simulink model "WindFarmGFMControl"  (R2025b)
settings: Solver=VariableStepAuto  StartTime=0.0  StopTime=Tsim  FixedStep=Ts  MaxStep=1  MinStep=Ts  RelTol=1e-3
PreLoadFcn:
  | run('WindFarmGFMControlParameters.m')
undefined symbols (not defined in the file): DiscIntNeverNeededParam, feeder, frt, gGFM, grid, line, loads, lvrt, mGFM, pmsm, time, Ts, windController, windTransformer, windTurbine
libraries: ee_lib x21, nesl_utility x14, eeGeneralControl x4, fl_lib x3, eeTransforms x2, eePowerMeasurement x1, eeSinusoidalMeasurementV2 x1
(part 2 of 2)

== system WindFarmGFMControl/Loads/CB1 ==
  Input : Inport
  Circuit Breaker Step off3 : ee_lib/Switches & Breakers/Circuit Breaker (Three-Phase)  R_closed=0.001 Ohm  G_open=1e-4 1/Ohm  threshold=0.5 V  breaker_behavior=ee.enum.switches.breakerBehavior.zeroCrossingDisable
      settings: InternalSimscapePortConfiguration="{\"Bottom\":[],\"Left\":[{\"id\":\"vT\",\"label\":\"vT\",\"type\":\"input\"},{\"id\":\"N1\",\"label\":\"~1\",\"type\":\"foundation.electrical.three_phase\"}],\"Right\":[{\"id\":\"N2\",\"label\":\"~2\",\"type\":\"foundation.electrical.three_phase\"}],\"Top\":[]}"
  Simulink-PS Converter3 : nesl_utility/Simulink-PS Converter  PhysicalDomain=network_engine_domain  SubClassName=ps_input  LeftPortType=input  RightPortType=output  PseudoPeriodic=off  Frequencies=[]  NoiseDistribution=none  NoiseParameters=[]  Unit=1  AffineConversion=off  FilteringAndDerivatives=zero  SimscapeFilterOrder=1  InputFilterTimeConstant=0.001  UdotUserProvided=1
  Conn2 : PMIOPort  Side=Left
  Conn1 : PMIOPort  Port=2  Side=Right
  wires:
  Input/1 -> Simulink-PS Converter3/1
  connections:
  Circuit Breaker Step off3/RConn1 -- Conn1/RConn1
  Circuit Breaker Step off3/LConn1 -- Simulink-PS Converter3/RConn1
  Circuit Breaker Step off3/LConn2 -- Conn2/RConn1

== system WindFarmGFMControl/PLL & Measurements/Measurement1 ==
  u : Inport
  Ig : Outport
  wires:
  u/1 -> Ig/1

== system WindFarmGFMControl/PLL & Measurements/Measurement2 ==
  u : Inport
  Vg : Outport
  wires:
  u/1 -> Vg/1

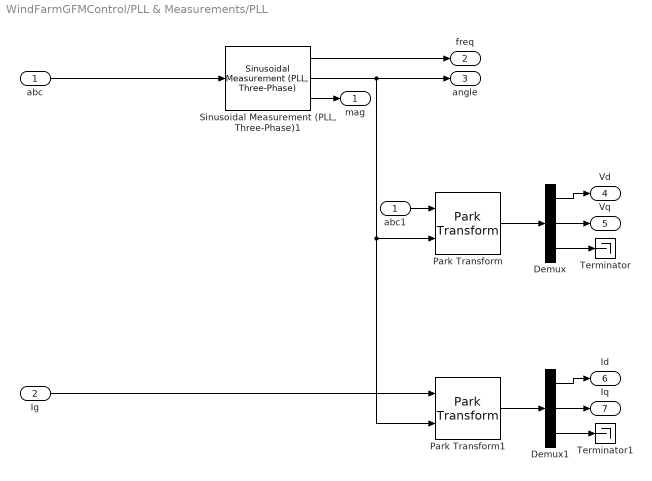
== system WindFarmGFMControl/PLL & Measurements/PLL ==
  abc : Inport
  Ig : Inport  Port=2
  Demux : Demux  Outputs=3
  Demux1 : Demux  Outputs=3
  Park Transform : eeTransforms/Park Transform  AxisAlignment=Q-axis  PowerInvariant=off
  Park Transform1 : eeTransforms/Park Transform  AxisAlignment=Q-axis  PowerInvariant=off
  "Sinusoidal Measurement (PLL, Three-Phase)1" : eeSinusoidalMeasurementV2/Sinusoidal Measurement (PLL, Three-Phase)  InputFilter=on  InputNormalization=off  Kp_LF=pll.kp  Ki_LF=pll.ki  F0=grid.frequency  Theta0=0  Ts=Ts
      settings: LibrarySourceBlock=|
      | ee_sl_lib/Measurements/Sinusoidal Measurement
      | (PLL, Three-Phase)
  Terminator : Terminator
  Terminator1 : Terminator
  abc1 : InportShadow
  mag : Outport
  freq : Outport  Port=2
  angle : Outport  Port=3
  Vd : Outport  Port=4
  Vq : Outport  Port=5
  Id : Outport  Port=6
  Iq : Outport  Port=7
  wires:
  Demux/3 -> Terminator/1
  Park Transform/1 -> Demux/1
  Demux/1 -> Vd/1
  Demux/2 -> Vq/1
  "Sinusoidal Measurement (PLL, Three-Phase)1"/3 -> mag/1
  "Sinusoidal Measurement (PLL, Three-Phase)1"/2 -> angle/1, Park Transform/2, Park Transform1/2
  Ig/1 -> Park Transform1/1
  Demux1/2 -> Iq/1
  Park Transform1/1 -> Demux1/1
  Demux1/1 -> Id/1
  Demux1/3 -> Terminator1/1
  abc1/1 -> Park Transform/1
  abc/1 -> "Sinusoidal Measurement (PLL, Three-Phase)1"/1
  "Sinusoidal Measurement (PLL, Three-Phase)1"/1 -> freq/1

== system WindFarmGFMControl/Wind Farm/CB2 ==
  Input : Inport
  Circuit Breaker Step off3 : ee_lib/Switches & Breakers/Circuit Breaker (Three-Phase)  R_closed=0.001 Ohm  G_open=1e-4 1/Ohm  threshold=0.5 V  breaker_behavior=ee.enum.switches.breakerBehavior.zeroCrossingDisable
      settings: InternalSimscapePortConfiguration="{\"Bottom\":[],\"Left\":[{\"id\":\"vT\",\"label\":\"vT\",\"type\":\"input\"},{\"id\":\"N1\",\"label\":\"~1\",\"type\":\"foundation.electrical.three_phase\"}],\"Right\":[{\"id\":\"N2\",\"label\":\"~2\",\"type\":\"foundation.electrical.three_phase\"}],\"Top\":[]}"
  Simulink-PS Converter3 : nesl_utility/Simulink-PS Converter  PhysicalDomain=network_engine_domain  SubClassName=ps_input  LeftPortType=input  RightPortType=output  PseudoPeriodic=off  Frequencies=[]  NoiseDistribution=none  NoiseParameters=[]  Unit=1  AffineConversion=off  FilteringAndDerivatives=zero  SimscapeFilterOrder=1  InputFilterTimeConstant=0.001  UdotUserProvided=1
  Conn2 : PMIOPort  Side=Left
  Conn1 : PMIOPort  Port=2  Side=Right
  wires:
  Input/1 -> Simulink-PS Converter3/1
  connections:
  Circuit Breaker Step off3/RConn1 -- Conn1/RConn1
  Circuit Breaker Step off3/LConn1 -- Simulink-PS Converter3/RConn1
  Circuit Breaker Step off3/LConn2 -- Conn2/RConn1

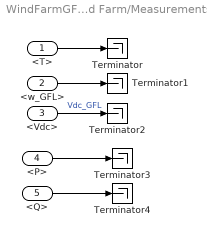
== system WindFarmGFMControl/Wind Farm/Measurements ==
  <T> : Inport
  <w_GFL> : Inport  Port=2
  <Vdc> : Inport  Port=3
  <P> : Inport  Port=4
  <Q> : Inport  Port=5
  Terminator{,1..4} (5 alike) : Terminator
  wires:
  <Vdc>/1 -> Terminator2/1  "Vdc_GFL"
  <Q>/1 -> Terminator4/1
  <w_GFL>/1 -> Terminator1/1
  <T>/1 -> Terminator/1
  <P>/1 -> Terminator3/1

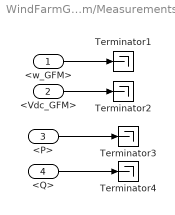
== system WindFarmGFMControl/Wind Farm/Measurements1 ==
  <w_GFM> : Inport
  <Vdc_GFM> : Inport  Port=2
  <P> : Inport  Port=3
  <Q> : Inport  Port=4
  Terminator{1..4} (4 alike) : Terminator
  wires:
  <P>/1 -> Terminator3/1
  <w_GFM>/1 -> Terminator1/1
  <Q>/1 -> Terminator4/1
  <Vdc_GFM>/1 -> Terminator2/1

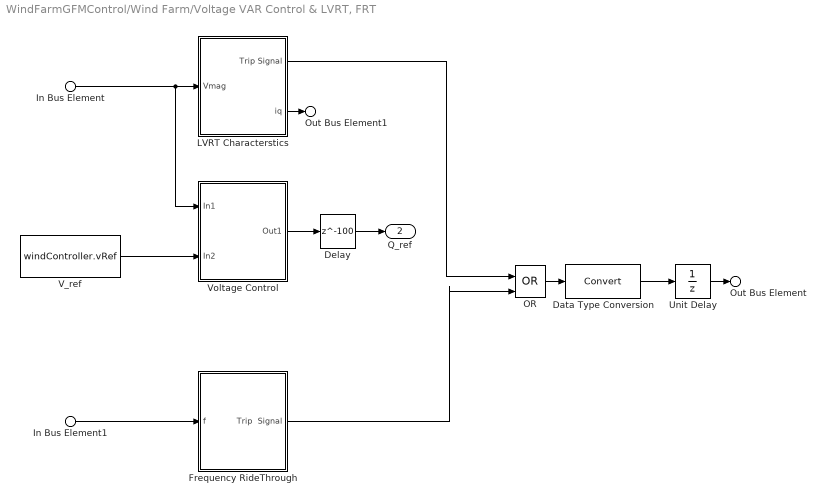
== system WindFarmGFMControl/Wind Farm/Voltage VAR Control & LVRT, FRT ==
  In Bus Element : Inport  PortName=Vbus  Element=Vmag
  In Bus Element1 : Inport  PortName=Vbus  Element=w
  Data Type Conversion : DataTypeConversion  RndMeth=Nearest  SaturateOnIntegerOverflow=off
  Delay : Delay  DelayLength=100
  Frequency RideThrough : Subsystem
  LVRT Characterstics : Subsystem
  OR : Logic  Operator=OR  IconShape=distinctive  AllPortsSameDT=off  OutDataTypeStr=boolean
  Unit Delay : UnitDelay  SampleTime=-1  HasFrameUpgradeWarning=on
  V_ref : Constant  Value=windController.vRef  SampleTime=Ts
  Voltage Control : Subsystem
  Out Bus Element : Outport  PortName=LVRT  Element=breaker
  Out Bus Element1 : Outport  PortName=LVRT  Element=iq
  Q_ref : Outport  Port=2
  wires:
  In Bus Element/1 -> LVRT Characterstics/1(Vmag), Voltage Control/1(In1)
  LVRT Characterstics/2(iq) -> Out Bus Element1/1
  V_ref/1 -> Voltage Control/2(In2)
  Voltage Control/1(Out1) -> Delay/1
  OR/1 -> Data Type Conversion/1
  LVRT Characterstics/1(Trip Signal) -> OR/1
  In Bus Element1/1 -> Frequency RideThrough/1(f)
  Data Type Conversion/1 -> Unit Delay/1
  Frequency RideThrough/1(Trip  Signal) -> OR/2
  Unit Delay/1 -> Out Bus Element/1
  Delay/1 -> Q_ref/1

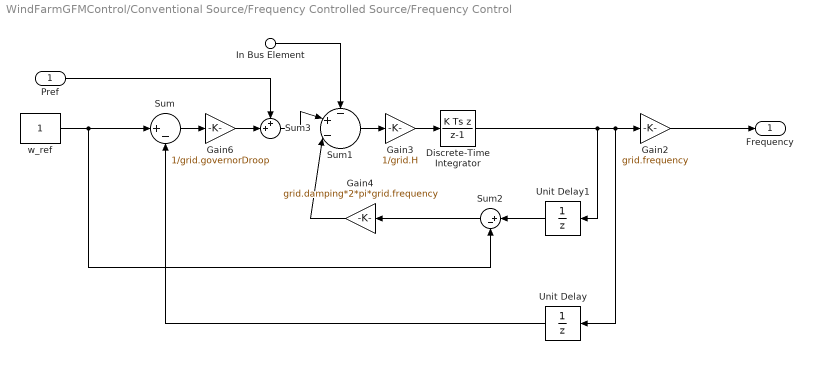
== system WindFarmGFMControl/Conventional Source/Frequency Controlled Source/Frequency Control ==
  Pref : Inport
  In Bus Element : Inport  Port=2  PortName=Grid  Element=Pe
  Discrete-Time Integrator : DiscreteIntegrator  IntegratorMethod=Integration: Backward Euler  InitialCondition=1  SampleTime=Ts  LimitOutput=on  UpperSaturationLimit=1.1  LowerSaturationLimit=0.9  ICPrevOutput=DiscIntNeverNeededParam  ICPrevScaledInput=DiscIntNeverNeededParam
  Gain2 : Gain  Gain=grid.frequency
  Gain3 : Gain  Gain=1/grid.H
  Gain4 : Gain  Gain=grid.damping*2*pi*grid.frequency
  Gain6 : Gain  Gain=1/grid.governorDroop
  Sum : Sum  Inputs=|+-
  Sum1 : Sum  Inputs=-+-|
  Sum2 : Sum  Inputs=|+-
  Sum3 : Sum  Inputs=++|
  Unit Delay : UnitDelay  InitialCondition=1  SampleTime=grid.sensorTime  HasFrameUpgradeWarning=on
  Unit Delay1 : UnitDelay  InitialCondition=1  SampleTime=grid.sensorTime  HasFrameUpgradeWarning=on
  w_ref : Constant
  Frequency : Outport
  wires:
  Sum3/1 -> Sum1/2
  w_ref/1 -> Sum2/2, Sum/1
  Sum1/1 -> Gain3/1
  Gain3/1 -> Discrete-Time Integrator/1
  Gain6/1 -> Sum3/2
  Gain2/1 -> Frequency/1
  Sum2/1 -> Gain4/1
  Sum/1 -> Gain6/1
  Pref/1 -> Sum3/1
  Gain4/1 -> Sum1/3
  In Bus Element/1 -> Sum1/1
  Discrete-Time Integrator/1 -> Unit Delay1/1, Unit Delay/1, Gain2/1
  Unit Delay/1 -> Sum/2
  Unit Delay1/1 -> Sum2/1

== system WindFarmGFMControl/Wind Farm/Voltage VAR Control & LVRT, FRT/Frequency RideThrough ==
  f : Inport
  Avoid Operation : Subsystem
  Discrete-Time Integrator1 : DiscreteIntegrator  ExternalReset=either  SampleTime=Ts  ICPrevOutput=DiscIntNeverNeededParam  ICPrevScaledInput=DiscIntNeverNeededParam
  Duration of f<fth : Lookup_n-D  NumberOfTableDimensions=1  BreakpointsForDimension1=(1+[-0.021,-0.02,0.02,0.021])*grid.frequency  Table=[1,0,0,1]  InterpMethod=Flat  InternalRulePriority=Speed  RndMeth=Simplest
  Frequency vs Trip time : Lookup_n-D  NumberOfTableDimensions=1  BreakpointsForDimension1=frt.frequency  Table=frt.time  InterpMethod=Flat  InternalRulePriority=Speed  RndMeth=Simplest
  GreaterThan : RelationalOperator  Operator=>  OutDataTypeStr=boolean  RndMeth=Simplest  InputSameDT=off
  Trip  Signal : Outport
  wires:
  Discrete-Time Integrator1/1 -> GreaterThan/1
  Frequency vs Trip time/1 -> GreaterThan/2
  GreaterThan/1 -> Trip  Signal/1
  Duration of f<fth/1 -> Discrete-Time Integrator1/2, Discrete-Time Integrator1/1
  Avoid Operation/1(f) -> Duration of f<fth/1, Frequency vs Trip time/1
  f/1 -> Avoid Operation/1(f_in)

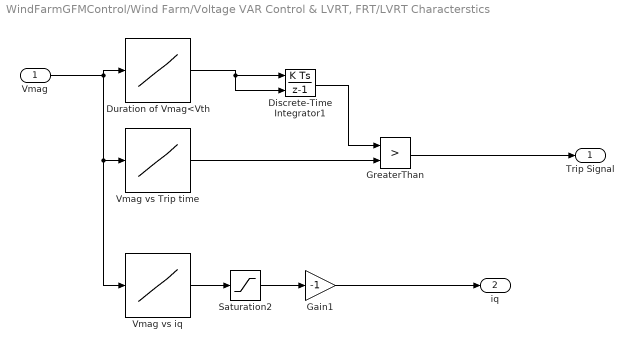
== system WindFarmGFMControl/Wind Farm/Voltage VAR Control & LVRT, FRT/LVRT Characterstics ==
  Vmag : Inport
  Discrete-Time Integrator1 : DiscreteIntegrator  ExternalReset=either  SampleTime=Ts  ICPrevOutput=DiscIntNeverNeededParam  ICPrevScaledInput=DiscIntNeverNeededParam
  Duration of Vmag<Vth : Lookup_n-D  NumberOfTableDimensions=1  BreakpointsForDimension1=[0,.9,0.91,1.2]  Table=[1,1,0,0]  InterpMethod=Flat  InternalRulePriority=Speed  RndMeth=Simplest
  Gain1 : Gain  Gain=-1
  GreaterThan : RelationalOperator  Operator=>  OutDataTypeStr=boolean  RndMeth=Simplest  InputSameDT=off
  Saturation2 : Saturate  UpperLimit=1/8  LowerLimit=-1
  Vmag vs Trip time : Lookup_n-D  NumberOfTableDimensions=1  BreakpointsForDimension1=lvrt.voltage  Table=lvrt.time  InterpMethod=Flat  InternalRulePriority=Speed  RndMeth=Simplest
  Vmag vs iq : Lookup_n-D  NumberOfTableDimensions=1  BreakpointsForDimension1=lvrt.voltageiq  Table=lvrt.iq  InternalRulePriority=Speed  RndMeth=Simplest
  Trip Signal : Outport
  iq : Outport  Port=2
  wires:
  Duration of Vmag<Vth/1 -> Discrete-Time Integrator1/2, Discrete-Time Integrator1/1
  GreaterThan/1 -> Trip Signal/1
  Discrete-Time Integrator1/1 -> GreaterThan/1
  Vmag vs Trip time/1 -> GreaterThan/2
  Vmag vs iq/1 -> Saturation2/1
  Gain1/1 -> iq/1
  Saturation2/1 -> Gain1/1
  Vmag/1 -> Vmag vs iq/1, Vmag vs Trip time/1, Duration of Vmag<Vth/1

== system WindFarmGFMControl/Wind Farm/Voltage VAR Control & LVRT, FRT/Voltage Control ==
  In1 : Inport
  In2 : Inport  Port=2
  Constant2 : Constant  Value=0
  Gain : Gain  Gain=windController.mv
  Sum2 : Sum  Inputs=|+-
  Switch1 : Switch  Threshold=.9  SaturateOnIntegerOverflow=off  InputSameDT=off
  Out1 : Outport
  wires:
  Gain/1 -> Out1/1
  Sum2/1 -> Switch1/1
  Switch1/1 -> Gain/1
  In1/1 -> Sum2/2, Switch1/2
  Constant2/1 -> Switch1/3
  In2/1 -> Sum2/1

== system WindFarmGFMControl/Wind Farm/Voltage VAR Control & LVRT, FRT/Frequency RideThrough/Avoid Operation ==
  f_in : Inport
  Constant : Constant  Value=grid.frequency  SampleTime=Ts
  Step : Step  Time=0.5  SampleTime=Ts
  Switch : Switch  Criteria=u2 > Threshold  SaturateOnIntegerOverflow=off  InputSameDT=off
  f : Outport
  wires:
  f_in/1 -> Switch/1
  Constant/1 -> Switch/3
  Step/1 -> Switch/2
  Switch/1 -> f/1
